simulink model "Frict3D_06_Ball_on_Balls"  (R2016a)
settings: Solver=ode23t  StartTime=0.0  StopTime=36  MaxStep=1e-2  RelTol=1e-4  AbsTol=1e-5
StartFcn:
  | tic;
StopFcn:
  | Elapsed_Sim_Time = toc;
  | disp(['Elapsed Sim Time = ' num2str(Elapsed_Sim_Time)]);
model workspace (MATLAB code in the model file):
  | % All units in meters
  | 
  | upper_ball.rad = 1;
  | lower_ball.rad = 0.2;
  | lower_ball.spacing = 0.5;
  | 
  | ballInput.mag = 80;
  | ballInput.filtconst = 0.4;
  | ballInput.period = 2;
  | ballInput.common.x = [0 1 0 -1 0 0 0  0 0 0 0  0 0];
  | ballInput.common.y = [0 0 0  0 0 1 0 -1 0 0 0  0 0];
  | ballInput.common.z = [0 0 0  0 0 0 0  0 0 1 0 -1 0];
  | 
  | ballInput.b1.x = [ballInput.common.x  0 0 0 0];
  | ballInput.b1.y = [ballInput.common.y  0 1 0 0];
  | ballInput.b2.x = [ballInput.common.x  0 0 0 0];
  | ballInput.b2.y = [ballInput.common.y  0 1 0 0];
  | ballInput.b3.x = [ballInput.common.x  0 0 0 0];
  | ballInput.b3.y = [ballInput.common.y  0 -1 0 0];
  | ballInput.b4.x = [ballInput.common.x  0 0 0 0];
  | ballInput.b4.y = [ballInput.common.y  0 -1 0 0];
  | ballInput.b1.z = [ballInput.common.z    0.5  0.5  0.5 0];
  | ballInput.b2.z = [ballInput.common.z   -0.5 -0.5 -0.5 0];
  | ballInput.b3.z = [ballInput.common.z    0.5  0.5  0.5 0];
  | ballInput.b4.z = [ballInput.common.z   -0.5 -0.5 -0.5 0];
undefined symbols (not defined in the file or in its folder): X, Y, Z
libraries: nesl_utility x13, simulink x12, sm_lib x12, Parts_Lib x5, Contact_Forces_Lib x4
CloseFcn:
  | try,close(h1_Frict3D_06_Ball_on_Balls),end
  | clear h1_Frict3D_06_Ball_on_Balls
  | 
  | clear logsout_Frict3D_06_Ball_on_Balls
  | clear simlog_Frict3D_06_Ball_on_Balls
Description:
  | Ball on Balls (3D)
  | 
  | Copyright 2015-2016 The MathWorks, Inc.
settings Model: Creator=smiller  LastModifiedBy=smiller
settings DataIOCC: SaveFormat=Array  SignalLoggingName=logsout_Frict3D_06_Ball_on_Balls
settings DebuggingCC: AlgebraicLoopMsg=error  SolverPrmCheckMsg=warning  UnconnectedOutputMsg=none  AllowSymbolicDim=off
settings HardwareCC: ProdBitPerPointer=32  ProdLargestAtomicFloat=None  ProdIntDivRoundTo=Undefined  ProdEndianess=Unspecified  ProdWordSize=32  ProdHWDeviceType=32-bit Generic
settings ModelReferenceCC: PropagateSignalLabelsOutOfModel=off
settings ConfigComp: CovModelRefEnable=Off  CovSFcnEnable=off
settings SimscapeCC: SimscapeLogType=all  SimscapeLogSimulationStatistics=on  SimscapeLogName=simlog_Frict3D_06_Ball_on_Balls  SimscapeLogLimitData=off  SimscapeLogDataHistory=10000
settings ConfigurationSet: Description=SimMechanics 2G
settings ExplorerConfigSet: InternalSimMechanicsExplorerSettings="<ExplorerConfiguration><canonicalview>default</canonicalview><AnimationSetting><BasePlaybackSpeed>1.0</BasePlaybackSpeed><PlaybackSpeedFactor>4.0</PlaybackSpeedFactor></AnimationSetting><TilePanel><TileInfo><Tiles Columns=\"1\" Count=\"1\" Rows=\"1\"><Column Left=\"2\" Weight=\"1\"/><Column Left=\"817\"/><Row Top=\"2\" Weight=\"1\"/><Row Top=\"877\"/><Tile Height=\"1\" Width=\"1\" X=\"0\" Y=\"0\"/></Tiles></TileInfo><SceneInfo><SceneViewer><BGColor><R>0.93333333730697632</R><G>0.9529411792755127</G><B>0.9529411792755127</B></BGColor><Camera><Position><X>3.2298659111445884</X><Y>-3.2298659111445884</Y><Z>4.1548559094851951</Z></Position><Center><X>0</X><Y>0</Y><Z>0.92498999834060669</Z></Center><Up><X>-0.40824829046386307</X><Y>0.40824829046386307</Y><Z>0.81649658092772615</Z></Up><Left>-2.2273862600326537</Left><Right>2.2273862600326537</Right><Bottom>-2.2504773259162905</Bottom><Top>2.2504773259162905</Top></Camera></SceneViewer></SceneInfo></TilePanel></ExplorerConfiguration>"

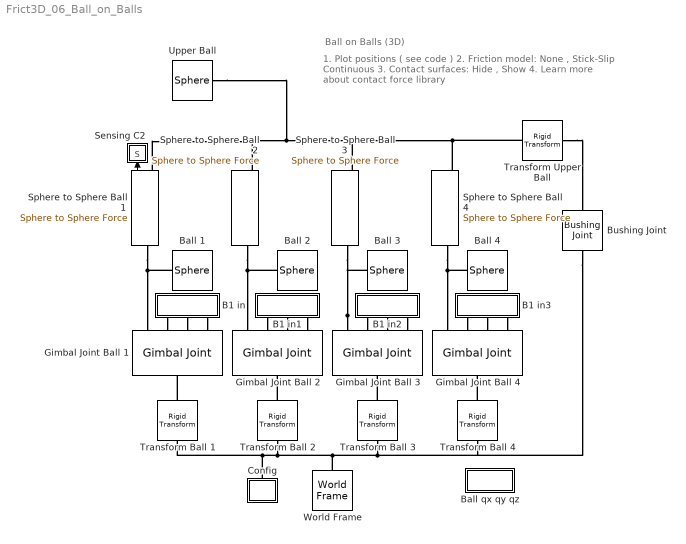
== system Frict3D_06_Ball_on_Balls ==
  note: 1. Plot positions ( see code )
      | 2. Friction model: None , Stick-Slip Continuous
      | 3. Contact surfaces: Hide , Show
      | 4. Learn more about contact force library
  note: Ball on Balls (3D)
  B1 in : Subsystem
  B1 in1 : Subsystem
  B1 in2 : Subsystem
  B1 in3 : Subsystem
  Ball {1..4} (4 alike) : Parts_Lib/Sphere  Tag=CustomStyle  sph_radius=lower_ball.rad  sph_density=1000  sph_color=blue  sph_opacity=1  mark_type=Rings on center planes  arc_width=[40 50]  arc_angle=60  ring_width=5  ring_irad=0.95  mark_color=axes  mark_opacity=1  ring_opacity=0  arc_opacity=0
  Ball qx qy qz : Subsystem
  Bushing Joint : sm_lib/Joints/Bushing Joint  SenseConstraintForce=off  SenseConstraintForceX=off  SenseConstraintForceY=off  SenseConstraintForceZ=off  SenseConstraintTorque=off  SenseConstraintTorqueX=off  SenseConstraintTorqueY=off  SenseConstraintTorqueZ=off  SenseTotalForce=off  SenseTotalForceX=off  SenseTotalForceY=off  SenseTotalForceZ=off  SenseTotalTorque=off  SenseTotalTorqueX=off  SenseTotalTorqueY=off  SenseTotalTorqueZ=off  CompositeWrenchDir=FollowerOnBase  CompositeWrenchFrame=BaseFrame  PxEquilibriumPosition=0  PxEquilibriumPositionUnits=m  PxSpringStiffness=0  PxSpringStiffnessUnits=N/m  PxDampingCoefficient=0  PxDampingCoefficientUnits=N/(m/s)  PxTorqueActuationMode=NoTorque  PxMotionActuationMode=ComputedMotion  PxSensePosition=off  PxSenseVelocity=off  PxSenseAcceleration=off  PxSenseTorqueForce=off  PxPositionTargetSpecify=off  PxPositionTargetPriority=High  PxPositionTargetValue=0  PxPositionTargetValueUnits=m  PxVelocityTargetSpecify=off  PxVelocityTargetPriority=High  PxVelocityTargetValue=0  PxVelocityTargetValueUnits=m/s  PyEquilibriumPosition=0  PyEquilibriumPositionUnits=m  PySpringStiffness=0  PySpringStiffnessUnits=N/m  PyDampingCoefficient=0  PyDampingCoefficientUnits=N/(m/s)  PyTorqueActuationMode=NoTorque  PyMotionActuationMode=ComputedMotion  PySensePosition=off  PySenseVelocity=off  PySenseAcceleration=off  PySenseTorqueForce=off  PyPositionTargetSpecify=off  PyPositionTargetPriority=High  PyPositionTargetValue=0  PyPositionTargetValueUnits=m  PyVelocityTargetSpecify=off  PyVelocityTargetPriority=High  PyVelocityTargetValue=0  PyVelocityTargetValueUnits=m/s  PzEquilibriumPosition=0  PzEquilibriumPositionUnits=m  PzSpringStiffness=0  PzSpringStiffnessUnits=N/m  PzDampingCoefficient=0  PzDampingCoefficientUnits=N/(m/s)  PzTorqueActuationMode=NoTorque  PzMotionActuationMode=ComputedMotion  PzSensePosition=off  PzSenseVelocity=off  PzSenseAcceleration=off  PzSenseTorqueForce=off  PzPositionTargetSpecify=on  PzPositionTargetPriority=High  PzPositionTargetValue=2  PzPositionTargetValueUnits=m  PzVelocityTargetSpecify=off  PzVelocityTargetPriority=High  PzVelocityTargetValue=0  PzVelocityTargetValueUnits=m/s  RxEquilibriumPosition=0  RxEquilibriumPositionUnits=deg  RxSpringStiffness=0  RxSpringStiffnessUnits=N*m/deg  RxDampingCoefficient=0  RxDampingCoefficientUnits=N*m/(deg/s)  RxTorqueActuationMode=NoTorque  RxMotionActuationMode=ComputedMotion  RxSensePosition=off  RxSenseVelocity=off  RxSenseAcceleration=off  RxSenseTorqueForce=off  RxPositionTargetSpecify=off  RxPositionTargetPriority=High  RxPositionTargetValue=0  RxPositionTargetValueUnits=deg  RxVelocityTargetSpecify=off  RxVelocityTargetPriority=High  RxVelocityTargetValue=0  RxVelocityTargetValueUnits=deg/s  RyEquilibriumPosition=0  RyEquilibriumPositionUnits=deg  RySpringStiffness=0  RySpringStiffnessUnits=N*m/deg  RyDampingCoefficient=0  RyDampingCoefficientUnits=N*m/(deg/s)  RyTorqueActuationMode=NoTorque  RyMotionActuationMode=ComputedMotion  RySensePosition=off  RySenseVelocity=off  RySenseAcceleration=off  RySenseTorqueForce=off  RyPositionTargetSpecify=off  RyPositionTargetPriority=High  RyPositionTargetValue=0  RyPositionTargetValueUnits=deg  RyVelocityTargetSpecify=off  RyVelocityTargetPriority=High  RyVelocityTargetValue=0  RyVelocityTargetValueUnits=deg/s  RzEquilibriumPosition=0  RzEquilibriumPositionUnits=deg  RzSpringStiffness=0  RzSpringStiffnessUnits=N*m/deg  RzDampingCoefficient=0  RzDampingCoefficientUnits=N*m/(deg/s)  RzTorqueActuationMode=NoTorque  RzMotionActuationMode=ComputedMotion  RzSensePosition=off  RzSenseVelocity=off  RzSenseAcceleration=off  RzSenseTorqueForce=off  RzPositionTargetSpecify=on  RzPositionTargetPriority=High  RzPositionTargetValue=0  RzPositionTargetValueUnits=deg  RzVelocityTargetSpecify=off  RzVelocityTargetPriority=High  RzVelocityTargetValue=0  RzVelocityTargetValueUnits=deg/s
  Config : Subsystem
  Gimbal Joint Ball {1..4} (4 alike) : sm_lib/Joints/Gimbal Joint  SenseConstraintForce=off  SenseConstraintForceX=off  SenseConstraintForceY=off  SenseConstraintForceZ=off  SenseConstraintTorque=off  SenseConstraintTorqueX=off  SenseConstraintTorqueY=off  SenseConstraintTorqueZ=off  SenseTotalForce=off  SenseTotalForceX=off  SenseTotalForceY=off  SenseTotalForceZ=off  SenseTotalTorque=off  SenseTotalTorqueX=off  SenseTotalTorqueY=off  SenseTotalTorqueZ=off  CompositeWrenchDir=FollowerOnBase  CompositeWrenchFrame=BaseFrame  RxEquilibriumPosition=0  RxEquilibriumPositionUnits=deg  RxSpringStiffness=0  RxSpringStiffnessUnits=N*m/deg  RxDampingCoefficient=0  RxDampingCoefficientUnits=N*m/(deg/s)  RxTorqueActuationMode=ComputedTorque  RxMotionActuationMode=InputMotion  RxSensePosition=off  RxSenseVelocity=off  RxSenseAcceleration=off  RxSenseTorqueForce=off  RxPositionTargetSpecify=off  RxPositionTargetPriority=High  RxPositionTargetValue=0  RxPositionTargetValueUnits=deg  RxVelocityTargetSpecify=off  RxVelocityTargetPriority=High  RxVelocityTargetValue=0  RxVelocityTargetValueUnits=deg/s  RyEquilibriumPosition=0  RyEquilibriumPositionUnits=deg  RySpringStiffness=0  RySpringStiffnessUnits=N*m/deg  RyDampingCoefficient=0  RyDampingCoefficientUnits=N*m/(deg/s)  RyTorqueActuationMode=ComputedTorque  RyMotionActuationMode=InputMotion  RySensePosition=off  RySenseVelocity=off  RySenseAcceleration=off  RySenseTorqueForce=off  RyPositionTargetSpecify=off  RyPositionTargetPriority=High  RyPositionTargetValue=0  RyPositionTargetValueUnits=deg  RyVelocityTargetSpecify=off  RyVelocityTargetPriority=High  RyVelocityTargetValue=0  RyVelocityTargetValueUnits=deg/s  RzEquilibriumPosition=0  RzEquilibriumPositionUnits=deg  RzSpringStiffness=0  RzSpringStiffnessUnits=N*m/deg  RzDampingCoefficient=0  RzDampingCoefficientUnits=N*m/(deg/s)  RzTorqueActuationMode=ComputedTorque  RzMotionActuationMode=InputMotion  RzSensePosition=off  RzSenseVelocity=off  RzSenseAcceleration=off  RzSenseTorqueForce=off  RzPositionTargetSpecify=off  RzPositionTargetPriority=High  RzPositionTargetValue=0  RzPositionTargetValueUnits=deg  RzVelocityTargetSpecify=off  RzVelocityTargetPriority=High  RzVelocityTargetValue=0  RzVelocityTargetValueUnits=deg/s
  Sensing C2 : Subsystem
  Sphere to Sphere Ball {1..4} (4 alike) : Contact_Forces_Lib/3D/Sphere to Sphere Force  sphB_rad=upper_ball.rad  sphF_rad=lower_ball.rad  force_law=Linear  k_contact=1e7  b_contact=1e5  pen_full_damp_F=1e-4  pen_exponent=1  custom_param_1=1  custom_param_2=1  friction_law=Stick-Slip Continuous  mu_kinetic=0.5  mu_static=0.7  v_thr=0.001  vis_on=off  vis_opc_en=0  vis_clr=[0.9 0.2 0.2]  vis_opc=0.7
  Transform Ball 1 : sm_lib/Frames and Transforms/Rigid Transform  TranslationMethod=Cartesian  TranslationLengthUnit=m  TranslationStandardAxis=+Z  TranslationStandardOffset=0  TranslationCartesianOffset=[1 1 0]*lower_ball.spacing  TranslationROffset=0  TranslationROffsetUnits=m  TranslationZOffset=0  TranslationZOffsetUnits=m  TranslationThetaOffset=0  TranslationThetaOffsetUnits=deg  RotationMethod=None  RotationAngleUnits=deg  RotationStandardAxis=+Z  RotationAngle=0.0  RotationArbitraryAxis=[0 0 1]  FollAlignAxisA=+X  BaseAlignAxisA=+Y  FollAlignAxisB=+Y  BaseAlignAxisB=+Z  RotationSequenceAxes=FollowerAxes  RotationSequence=XYX  RotationSequenceAngles=[0 0 0]  RotationSequenceAnglesUnits=deg  RotationMatrix=[1 0 0; 0 1 0; 0 0 1]
  Transform Ball 2 : sm_lib/Frames and Transforms/Rigid Transform  TranslationMethod=Cartesian  TranslationLengthUnit=m  TranslationStandardAxis=+Z  TranslationStandardOffset=0  TranslationCartesianOffset=[-1 1 0]*lower_ball.spacing  TranslationROffset=0  TranslationROffsetUnits=m  TranslationZOffset=0  TranslationZOffsetUnits=m  TranslationThetaOffset=0  TranslationThetaOffsetUnits=deg  RotationMethod=None  RotationAngleUnits=deg  RotationStandardAxis=+Z  RotationAngle=0.0  RotationArbitraryAxis=[0 0 1]  FollAlignAxisA=+X  BaseAlignAxisA=+Y  FollAlignAxisB=+Y  BaseAlignAxisB=+Z  RotationSequenceAxes=FollowerAxes  RotationSequence=XYX  RotationSequenceAngles=[0 0 0]  RotationSequenceAnglesUnits=deg  RotationMatrix=[1 0 0; 0 1 0; 0 0 1]
  Transform Ball 3 : sm_lib/Frames and Transforms/Rigid Transform  TranslationMethod=Cartesian  TranslationLengthUnit=m  TranslationStandardAxis=+Z  TranslationStandardOffset=0  TranslationCartesianOffset=[-1 -1 0]*lower_ball.spacing  TranslationROffset=0  TranslationROffsetUnits=m  TranslationZOffset=0  TranslationZOffsetUnits=m  TranslationThetaOffset=0  TranslationThetaOffsetUnits=deg  RotationMethod=None  RotationAngleUnits=deg  RotationStandardAxis=+Z  RotationAngle=0.0  RotationArbitraryAxis=[0 0 1]  FollAlignAxisA=+X  BaseAlignAxisA=+Y  FollAlignAxisB=+Y  BaseAlignAxisB=+Z  RotationSequenceAxes=FollowerAxes  RotationSequence=XYX  RotationSequenceAngles=[0 0 0]  RotationSequenceAnglesUnits=deg  RotationMatrix=[1 0 0; 0 1 0; 0 0 1]
  Transform Ball 4 : sm_lib/Frames and Transforms/Rigid Transform  TranslationMethod=Cartesian  TranslationLengthUnit=m  TranslationStandardAxis=+Z  TranslationStandardOffset=0  TranslationCartesianOffset=[1 -1 0]*lower_ball.spacing  TranslationROffset=0  TranslationROffsetUnits=m  TranslationZOffset=0  TranslationZOffsetUnits=m  TranslationThetaOffset=0  TranslationThetaOffsetUnits=deg  RotationMethod=None  RotationAngleUnits=deg  RotationStandardAxis=+Z  RotationAngle=0.0  RotationArbitraryAxis=[0 0 1]  FollAlignAxisA=+X  BaseAlignAxisA=+Y  FollAlignAxisB=+Y  BaseAlignAxisB=+Z  RotationSequenceAxes=FollowerAxes  RotationSequence=XYX  RotationSequenceAngles=[0 0 0]  RotationSequenceAnglesUnits=deg  RotationMatrix=[1 0 0; 0 1 0; 0 0 1]
  Transform Upper Ball : sm_lib/Frames and Transforms/Rigid Transform  TranslationMethod=None  TranslationLengthUnit=m  TranslationStandardAxis=+Z  TranslationStandardOffset=0  TranslationCartesianOffset=[0 0 0]  TranslationROffset=0  TranslationROffsetUnits=m  TranslationZOffset=0  TranslationZOffsetUnits=m  TranslationThetaOffset=0  TranslationThetaOffsetUnits=deg  RotationMethod=StandardAxis  RotationAngleUnits=deg  RotationStandardAxis=+X  RotationAngle=90.0  RotationArbitraryAxis=[0 0 1]  FollAlignAxisA=+X  BaseAlignAxisA=+Y  FollAlignAxisB=+Y  BaseAlignAxisB=+Z  RotationSequenceAxes=FollowerAxes  RotationSequence=XYX  RotationSequenceAngles=[0 0 0]  RotationSequenceAnglesUnits=deg  RotationMatrix=[1 0 0; 0 1 0; 0 0 1]
  Upper Ball : Parts_Lib/Sphere  Tag=CustomStyle  sph_radius=upper_ball.rad  sph_density=1000  sph_color=gray  sph_opacity=1  mark_type=Rings on center planes  arc_width=[40 50]  arc_angle=60  ring_width=5  ring_irad=0.95  mark_color=axes  mark_opacity=1  ring_opacity=0  arc_opacity=0
  World Frame : sm_lib/Frames and Transforms/World Frame
  wires:
  Sphere to Sphere Ball 1/1 -> Sensing C2/1(S)
  connections:
  World Frame/RConn1 -- Bushing Joint/LConn1 -- Transform Ball 4/RConn1 -- Transform Ball 3/RConn1 -- Transform Ball 1/RConn1 -- Config/LConn1 -- Transform Ball 2/RConn1
  Transform Ball 1/LConn1 -- Gimbal Joint Ball 1/RConn1
  Transform Ball 2/LConn1 -- Gimbal Joint Ball 2/RConn1
  Transform Ball 3/LConn1 -- Gimbal Joint Ball 3/RConn1
  Transform Ball 4/LConn1 -- Gimbal Joint Ball 4/RConn1
  B1 in/RConn1 -- Gimbal Joint Ball 1/LConn2
  B1 in/RConn2 -- Gimbal Joint Ball 1/LConn3
  B1 in/RConn3 -- Gimbal Joint Ball 1/LConn4
  Ball 1/LConn1 -- Sphere to Sphere Ball 1/LConn1 -- Gimbal Joint Ball 1/LConn1
  Sphere to Sphere Ball 2/RConn1 -- Sphere to Sphere Ball 1/RConn1 -- Upper Ball/LConn1 -- Sphere to Sphere Ball 3/RConn1 -- Sphere to Sphere Ball 4/RConn1 -- Transform Upper Ball/RConn1
  Ball 2/LConn1 -- Sphere to Sphere Ball 2/LConn1 -- Gimbal Joint Ball 2/LConn1
  Gimbal Joint Ball 3/LConn1 -- Sphere to Sphere Ball 3/LConn1 -- Ball 3/LConn1
  Ball 4/LConn1 -- Sphere to Sphere Ball 4/LConn1 -- Gimbal Joint Ball 4/LConn1
  B1 in1/RConn1 -- Gimbal Joint Ball 2/LConn2
  B1 in1/RConn2 -- Gimbal Joint Ball 2/LConn3
  B1 in1/RConn3 -- Gimbal Joint Ball 2/LConn4
  B1 in2/RConn1 -- Gimbal Joint Ball 3/LConn2
  B1 in2/RConn2 -- Gimbal Joint Ball 3/LConn3
  B1 in2/RConn3 -- Gimbal Joint Ball 3/LConn4
  B1 in3/RConn1 -- Gimbal Joint Ball 4/LConn2
  B1 in3/RConn2 -- Gimbal Joint Ball 4/LConn3
  B1 in3/RConn3 -- Gimbal Joint Ball 4/LConn4
  Transform Upper Ball/LConn1 -- Bushing Joint/RConn1

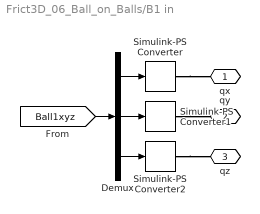
== system Frict3D_06_Ball_on_Balls/B1 in ==
  Demux : Demux  Outputs=3
  Simulink-PS Converter : nesl_utility/Simulink-PS Converter  PhysicalDomain=network_engine_domain  SubClassName=ps_input  LeftPortType=input  RightPortType=output  PseudoPeriodic=off  Frequencies=[]  NoiseDistribution=none  NoiseParameters=[]  Unit=deg  AffineConversion=off  InputFiltering=on  SimscapeFilterOrder=2  InputFilterTimeConstant=ballInput.filtconst  UdotUserProvided=1
  Simulink-PS Converter1 : nesl_utility/Simulink-PS Converter  PhysicalDomain=network_engine_domain  SubClassName=ps_input  LeftPortType=input  RightPortType=output  PseudoPeriodic=off  Frequencies=[]  NoiseDistribution=none  NoiseParameters=[]  Unit=deg  AffineConversion=off  InputFiltering=on  SimscapeFilterOrder=2  InputFilterTimeConstant=ballInput.filtconst  UdotUserProvided=1
  Simulink-PS Converter2 : nesl_utility/Simulink-PS Converter  PhysicalDomain=network_engine_domain  SubClassName=ps_input  LeftPortType=input  RightPortType=output  PseudoPeriodic=off  Frequencies=[]  NoiseDistribution=none  NoiseParameters=[]  Unit=deg  AffineConversion=off  InputFiltering=on  SimscapeFilterOrder=2  InputFilterTimeConstant=ballInput.filtconst  UdotUserProvided=1
  qx : PMIOPort  Port=1  Side=Right
  qy : PMIOPort  Port=2  Side=Right
  qz : PMIOPort  Port=3  Side=Right
  wires:
  Demux/3 -> Simulink-PS Converter2/1
  Demux/1 -> Simulink-PS Converter/1
  [Ball1xyz] -> Demux/1
  Demux/2 -> Simulink-PS Converter1/1
  connections:
  Simulink-PS Converter/RConn1 -- qx/RConn1
  Simulink-PS Converter1/RConn1 -- qy/RConn1
  Simulink-PS Converter2/RConn1 -- qz/RConn1

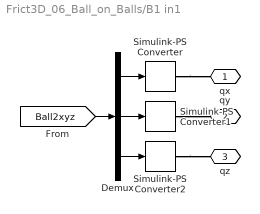
== system Frict3D_06_Ball_on_Balls/B1 in1 ==
  Demux : Demux  Outputs=3
  Simulink-PS Converter : nesl_utility/Simulink-PS Converter  PhysicalDomain=network_engine_domain  SubClassName=ps_input  LeftPortType=input  RightPortType=output  PseudoPeriodic=off  Frequencies=[]  NoiseDistribution=none  NoiseParameters=[]  Unit=deg  AffineConversion=off  InputFiltering=on  SimscapeFilterOrder=2  InputFilterTimeConstant=ballInput.filtconst  UdotUserProvided=1
  Simulink-PS Converter1 : nesl_utility/Simulink-PS Converter  PhysicalDomain=network_engine_domain  SubClassName=ps_input  LeftPortType=input  RightPortType=output  PseudoPeriodic=off  Frequencies=[]  NoiseDistribution=none  NoiseParameters=[]  Unit=deg  AffineConversion=off  InputFiltering=on  SimscapeFilterOrder=2  InputFilterTimeConstant=ballInput.filtconst  UdotUserProvided=1
  Simulink-PS Converter2 : nesl_utility/Simulink-PS Converter  PhysicalDomain=network_engine_domain  SubClassName=ps_input  LeftPortType=input  RightPortType=output  PseudoPeriodic=off  Frequencies=[]  NoiseDistribution=none  NoiseParameters=[]  Unit=deg  AffineConversion=off  InputFiltering=on  SimscapeFilterOrder=2  InputFilterTimeConstant=ballInput.filtconst  UdotUserProvided=1
  qx : PMIOPort  Port=1  Side=Right
  qy : PMIOPort  Port=2  Side=Right
  qz : PMIOPort  Port=3  Side=Right
  wires:
  Demux/2 -> Simulink-PS Converter1/1
  [Ball2xyz] -> Demux/1
  Demux/1 -> Simulink-PS Converter/1
  Demux/3 -> Simulink-PS Converter2/1
  connections:
  Simulink-PS Converter2/RConn1 -- qz/RConn1
  Simulink-PS Converter1/RConn1 -- qy/RConn1
  Simulink-PS Converter/RConn1 -- qx/RConn1

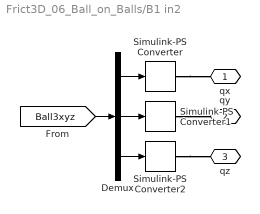
== system Frict3D_06_Ball_on_Balls/B1 in2 ==
  Demux : Demux  Outputs=3
  Simulink-PS Converter : nesl_utility/Simulink-PS Converter  PhysicalDomain=network_engine_domain  SubClassName=ps_input  LeftPortType=input  RightPortType=output  PseudoPeriodic=off  Frequencies=[]  NoiseDistribution=none  NoiseParameters=[]  Unit=deg  AffineConversion=off  InputFiltering=on  SimscapeFilterOrder=2  InputFilterTimeConstant=ballInput.filtconst  UdotUserProvided=1
  Simulink-PS Converter1 : nesl_utility/Simulink-PS Converter  PhysicalDomain=network_engine_domain  SubClassName=ps_input  LeftPortType=input  RightPortType=output  PseudoPeriodic=off  Frequencies=[]  NoiseDistribution=none  NoiseParameters=[]  Unit=deg  AffineConversion=off  InputFiltering=on  SimscapeFilterOrder=2  InputFilterTimeConstant=ballInput.filtconst  UdotUserProvided=1
  Simulink-PS Converter2 : nesl_utility/Simulink-PS Converter  PhysicalDomain=network_engine_domain  SubClassName=ps_input  LeftPortType=input  RightPortType=output  PseudoPeriodic=off  Frequencies=[]  NoiseDistribution=none  NoiseParameters=[]  Unit=deg  AffineConversion=off  InputFiltering=on  SimscapeFilterOrder=2  InputFilterTimeConstant=ballInput.filtconst  UdotUserProvided=1
  qx : PMIOPort  Port=1  Side=Right
  qy : PMIOPort  Port=2  Side=Right
  qz : PMIOPort  Port=3  Side=Right
  wires:
  Demux/3 -> Simulink-PS Converter2/1
  Demux/1 -> Simulink-PS Converter/1
  [Ball3xyz] -> Demux/1
  Demux/2 -> Simulink-PS Converter1/1
  connections:
  Simulink-PS Converter/RConn1 -- qx/RConn1
  Simulink-PS Converter1/RConn1 -- qy/RConn1
  Simulink-PS Converter2/RConn1 -- qz/RConn1

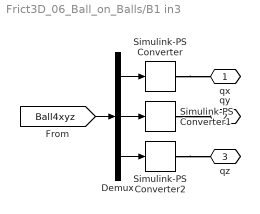
== system Frict3D_06_Ball_on_Balls/B1 in3 ==
  Demux : Demux  Outputs=3
  Simulink-PS Converter : nesl_utility/Simulink-PS Converter  PhysicalDomain=network_engine_domain  SubClassName=ps_input  LeftPortType=input  RightPortType=output  PseudoPeriodic=off  Frequencies=[]  NoiseDistribution=none  NoiseParameters=[]  Unit=deg  AffineConversion=off  InputFiltering=on  SimscapeFilterOrder=2  InputFilterTimeConstant=ballInput.filtconst  UdotUserProvided=1
  Simulink-PS Converter1 : nesl_utility/Simulink-PS Converter  PhysicalDomain=network_engine_domain  SubClassName=ps_input  LeftPortType=input  RightPortType=output  PseudoPeriodic=off  Frequencies=[]  NoiseDistribution=none  NoiseParameters=[]  Unit=deg  AffineConversion=off  InputFiltering=on  SimscapeFilterOrder=2  InputFilterTimeConstant=ballInput.filtconst  UdotUserProvided=1
  Simulink-PS Converter2 : nesl_utility/Simulink-PS Converter  PhysicalDomain=network_engine_domain  SubClassName=ps_input  LeftPortType=input  RightPortType=output  PseudoPeriodic=off  Frequencies=[]  NoiseDistribution=none  NoiseParameters=[]  Unit=deg  AffineConversion=off  InputFiltering=on  SimscapeFilterOrder=2  InputFilterTimeConstant=ballInput.filtconst  UdotUserProvided=1
  qx : PMIOPort  Port=1  Side=Right
  qy : PMIOPort  Port=2  Side=Right
  qz : PMIOPort  Port=3  Side=Right
  wires:
  Demux/2 -> Simulink-PS Converter1/1
  [Ball4xyz] -> Demux/1
  Demux/1 -> Simulink-PS Converter/1
  Demux/3 -> Simulink-PS Converter2/1
  connections:
  Simulink-PS Converter2/RConn1 -- qz/RConn1
  Simulink-PS Converter1/RConn1 -- qy/RConn1
  Simulink-PS Converter/RConn1 -- qx/RConn1

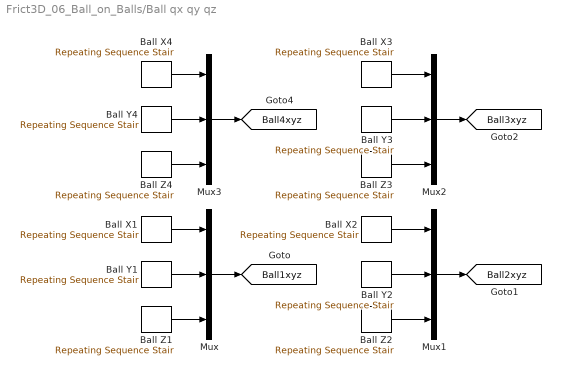
== system Frict3D_06_Ball_on_Balls/Ball qx qy qz ==
  Ball X1 : simulink/Sources/Repeating Sequence Stair  OutValues=ballInput.b1.x.'*ballInput.mag  tsamp=ballInput.period  OutMin=[]  OutMax=[]  OutDataTypeStr=double  OutputDataTypeScalingMode=double  OutDataType=fixdt(0,8)  ConRadixGroup=Best Precision: Vector-wise  OutScaling=2^-12
  Ball X2 : simulink/Sources/Repeating Sequence Stair  OutValues=ballInput.b2.x.'*ballInput.mag  tsamp=ballInput.period  OutMin=[]  OutMax=[]  OutDataTypeStr=double  OutputDataTypeScalingMode=double  OutDataType=fixdt(0,8)  ConRadixGroup=Best Precision: Vector-wise  OutScaling=2^-12
  Ball X3 : simulink/Sources/Repeating Sequence Stair  OutValues=ballInput.b3.x.'*ballInput.mag  tsamp=ballInput.period  OutMin=[]  OutMax=[]  OutDataTypeStr=double  OutputDataTypeScalingMode=double  OutDataType=fixdt(0,8)  ConRadixGroup=Best Precision: Vector-wise  OutScaling=2^-12
  Ball X4 : simulink/Sources/Repeating Sequence Stair  OutValues=ballInput.b4.x.'*ballInput.mag  tsamp=ballInput.period  OutMin=[]  OutMax=[]  OutDataTypeStr=double  OutputDataTypeScalingMode=double  OutDataType=fixdt(0,8)  ConRadixGroup=Best Precision: Vector-wise  OutScaling=2^-12
  Ball Y1 : simulink/Sources/Repeating Sequence Stair  OutValues=ballInput.b1.y.'*ballInput.mag  tsamp=ballInput.period  OutMin=[]  OutMax=[]  OutDataTypeStr=double  OutputDataTypeScalingMode=double  OutDataType=fixdt(0,8)  ConRadixGroup=Best Precision: Vector-wise  OutScaling=2^-12
  Ball Y2 : simulink/Sources/Repeating Sequence Stair  OutValues=ballInput.b2.y.'*ballInput.mag  tsamp=ballInput.period  OutMin=[]  OutMax=[]  OutDataTypeStr=double  OutputDataTypeScalingMode=double  OutDataType=fixdt(0,8)  ConRadixGroup=Best Precision: Vector-wise  OutScaling=2^-12
  Ball Y3 : simulink/Sources/Repeating Sequence Stair  OutValues=ballInput.b3.y.'*ballInput.mag  tsamp=ballInput.period  OutMin=[]  OutMax=[]  OutDataTypeStr=double  OutputDataTypeScalingMode=double  OutDataType=fixdt(0,8)  ConRadixGroup=Best Precision: Vector-wise  OutScaling=2^-12
  Ball Y4 : simulink/Sources/Repeating Sequence Stair  OutValues=ballInput.b4.y.'*ballInput.mag  tsamp=ballInput.period  OutMin=[]  OutMax=[]  OutDataTypeStr=double  OutputDataTypeScalingMode=double  OutDataType=fixdt(0,8)  ConRadixGroup=Best Precision: Vector-wise  OutScaling=2^-12
  Ball Z1 : simulink/Sources/Repeating Sequence Stair  OutValues=ballInput.b1.z.'*ballInput.mag  tsamp=ballInput.period  OutMin=[]  OutMax=[]  OutDataTypeStr=double  OutputDataTypeScalingMode=double  OutDataType=fixdt(0,8)  ConRadixGroup=Best Precision: Vector-wise  OutScaling=2^-12
  Ball Z2 : simulink/Sources/Repeating Sequence Stair  OutValues=ballInput.b2.z.'*ballInput.mag  tsamp=ballInput.period  OutMin=[]  OutMax=[]  OutDataTypeStr=double  OutputDataTypeScalingMode=double  OutDataType=fixdt(0,8)  ConRadixGroup=Best Precision: Vector-wise  OutScaling=2^-12
  Ball Z3 : simulink/Sources/Repeating Sequence Stair  OutValues=ballInput.b3.z.'*ballInput.mag  tsamp=ballInput.period  OutMin=[]  OutMax=[]  OutDataTypeStr=double  OutputDataTypeScalingMode=double  OutDataType=fixdt(0,8)  ConRadixGroup=Best Precision: Vector-wise  OutScaling=2^-12
  Ball Z4 : simulink/Sources/Repeating Sequence Stair  OutValues=ballInput.b4.z.'*ballInput.mag  tsamp=ballInput.period  OutMin=[]  OutMax=[]  OutDataTypeStr=double  OutputDataTypeScalingMode=double  OutDataType=fixdt(0,8)  ConRadixGroup=Best Precision: Vector-wise  OutScaling=2^-12
  Mux{,1..3} (4 alike) : Mux  Inputs=3
  tag scope: Ball1xyz=global, Ball2xyz=global, Ball3xyz=global, Ball4xyz=global
  wires:
  Ball Y1/1 -> Mux/2
  Ball X1/1 -> Mux/1
  Ball Z1/1 -> Mux/3
  Mux/1 -> [Ball1xyz]
  Ball Y2/1 -> Mux1/2
  Ball X2/1 -> Mux1/1
  Ball Z2/1 -> Mux1/3
  Mux1/1 -> [Ball2xyz]
  Ball Y3/1 -> Mux2/2
  Ball X3/1 -> Mux2/1
  Ball Z3/1 -> Mux2/3
  Mux2/1 -> [Ball3xyz]
  Ball Y4/1 -> Mux3/2
  Ball X4/1 -> Mux3/1
  Ball Z4/1 -> Mux3/3
  Mux3/1 -> [Ball4xyz]

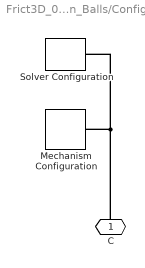
== system Frict3D_06_Ball_on_Balls/Config ==
  Mechanism Configuration : sm_lib/Utilities/Mechanism Configuration  UniformGravity=Constant  GravityVector=[0 0 -9.80665]  GravityUnits=m/s^2  LinearizationDelta=0.001
  Solver Configuration : nesl_utility/Solver Configuration  PhysicalDomain=network_engine_domain  SubClassName=solver  LeftPortType=input  RightPortType=generic  Accelerate=off  Tones=[]  Harmonics=[]  SimulateNoise=off  Profile=off  UseLocalSampling=off  EnableSwitchedLinearOptims=on  FrequencyDomain=off  UseCCode=off  RelTol=0.001  AbsTol=1e-06  MinStep=1e-09  ToWorkspace=off  RevertToSquareIcSolve=off  NumHomotopyIterations=100  PhasorMode=off  PhasorModeNumHarmonics=1  OverrideAbsTol=off  DoDC=off  ResidualTolerance=1e-09  UseLocalSolver=off  LocalSolverChoice=NE_BACKWARD_EULER_ADVANCER  LocalSolverSampleTime=0.001  DoFixedCost=off  MaxNonlinIter=3  MaxModeIter=2  LinearAlgebra=Sparse  DelaysMemoryBudget=1024  AutomaticFiltering=on  FilteringTimeConstant=0.001
  C : PMIOPort  Port=1  Side=Left
  connections:
  Solver Configuration/RConn1 -- C/RConn1 -- Mechanism Configuration/RConn1

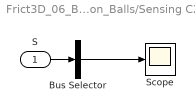
== system Frict3D_06_Ball_on_Balls/Sensing C2 ==
  S : Inport
  Bus Selector : BusSelector  OutputSignals=Frame Sep.dst  OutputAsBus=on
  Scope : Scope
  wires:
  Bus Selector/1 -> Scope/1
  S/1 -> Bus Selector/1
